simulink model "model"  (R2022b)
settings: Solver=VariableStepAuto  StartTime=0.0  StopTime=10.0  RelTol=1e-3
undefined symbols (not defined in the file or in its folder): jz, ke, ki, la, ra
settings Model: Creator=molsz  LastModifiedBy=molsz

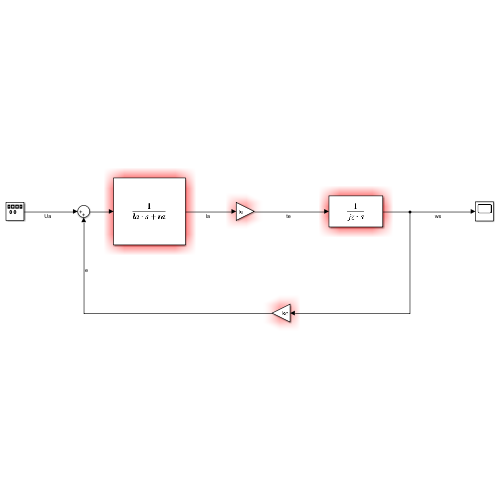
[thumbnail: Simulink's stored preview of the top-level diagram]
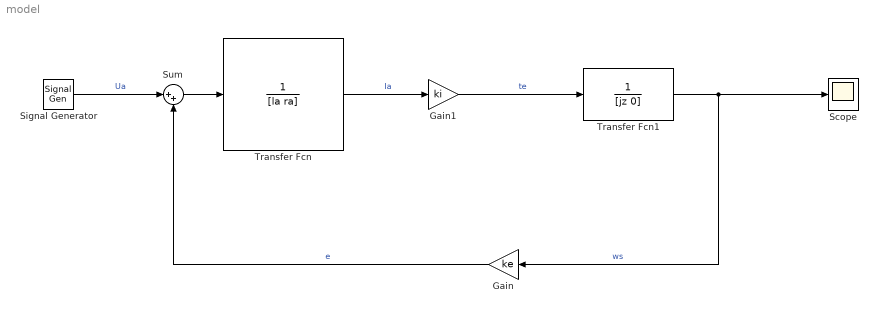
== system model ==
  Gain : Gain  Gain=ke
  Gain1 : Gain  Gain=ki
  Scope : Scope
  Signal Generator : SignalGenerator  Units=rad/sec
  Sum : Sum  Inputs=|++
  Transfer Fcn : TransferFcn  Denominator=[la ra]
  Transfer Fcn1 : TransferFcn  Denominator=[jz 0]
  wires:
  Sum/1 -> Transfer Fcn/1
  Signal Generator/1 -> Sum/1  "Ua"
  Gain/1 -> Sum/2  "e"
  Transfer Fcn/1 -> Gain1/1  "Ia"
  Gain1/1 -> Transfer Fcn1/1  "te"
  Transfer Fcn1/1 -> Gain/1, Scope/1  "ws"
